simulink model "oldMLpendubotSimulink"  (R2024b)
settings: Solver=FixedStepAuto  StartTime=0.0  StopTime=10  FixedStep=dt  RelTol=1e-3
InitFcn:
  | simpb_init
values from neighbouring files (symbols this model uses):
  dt = 0.01    [EKF_stateFNpb.m]    (also in downrighttest.m = 0.001; pendubot_lqr.m; simpb_init.m)
  eqb = [-pi/2;0;0;0]    [downrighttest.m]    (also in pendubot_lqr.m = [pi/2;0;0;0]; simpb_init.m = [pi/2;0;0;0])
  mNoise = diag([mvar,mvar])    [downrighttest.m]    (also in simpb_init.m)
  mvar = 1e-3    (= 0.001)    [downrighttest.m]    (also in simpb_init.m = 0.0001)
  pNoise = diag([pvar,pvar,pvar,pvar])    [downrighttest.m]    (also in simpb_init.m)
  pvar = 0    [downrighttest.m]    (also in simpb_init.m = 1e-06)
  Q = diag([15,15,1,1])    [downrighttest.m]    (also in pendubot_lqr.m = diag([10,10,1,1]); simpb_init.m = diag([150,250,100,200]))
  q1dref = interp1(t_ref, q1dref, t_sim, 'pchip')    [pendubot_lqr.m]    (also in simpb_init.m)
  q1ref = interp1(t_ref, q1ref, t_sim, 'pchip')    [pendubot_lqr.m]    (also in simpb_init.m)
  q2dref = interp1(t_ref, q2dref, t_sim, 'pchip')    [pendubot_lqr.m]    (also in simpb_init.m)
  q2ref = interp1(t_ref, q2ref, t_sim, 'pchip')    [pendubot_lqr.m]    (also in simpb_init.m)
  R = 50    [downrighttest.m]    (also in pendubot_lqr.m = 5; simpb_init.m)
  uref = interp1(t_ref, uref, t_sim, 'pchip')    [pendubot_lqr.m]    (also in simpb_init.m)
  x0 = [-pi/4;0;0;0]    [downrighttest.m]    (also in pendubot_lqr.m = [-pi/2;0;0;0])
libraries: sharedTrackingLibrary x1
settings Model: Creator=heeirthan  LastModifiedBy=heeirthan

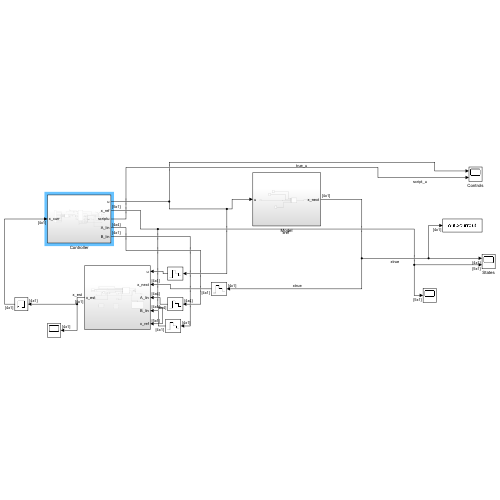
[thumbnail: Simulink's stored preview of the top-level diagram]
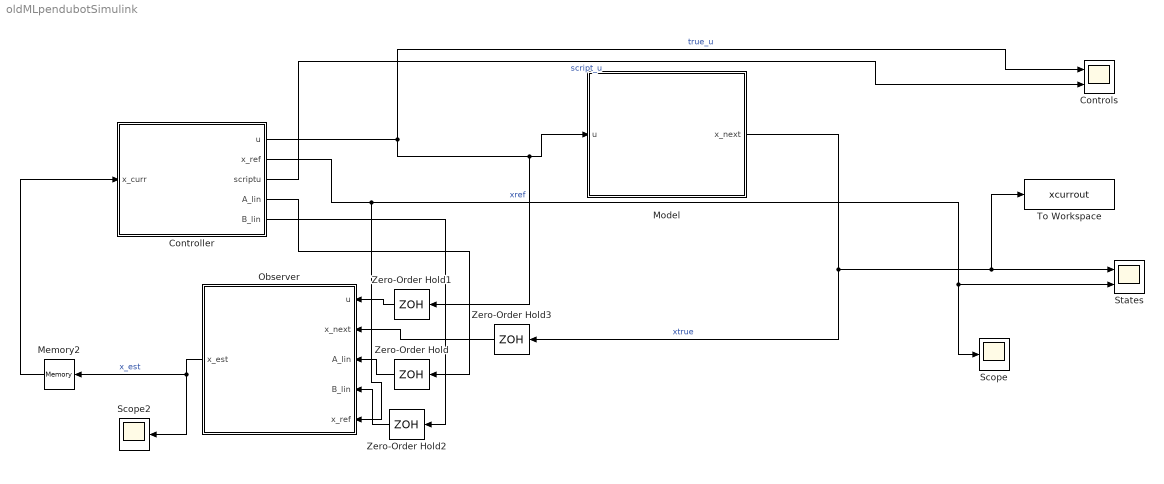
== system oldMLpendubotSimulink ==
  Controller : Subsystem
  Controls : Scope  NumInputPorts=2
  Memory2 : Memory  InitialCondition=x0
  Model : Subsystem
  Observer : Subsystem
  Scope : Scope
  Scope2 : Scope
  States : Scope  NumInputPorts=2
  To Workspace : ToWorkspace  VariableName=xcurrout  SaveFormat=Timeseries  SampleTime=-1
  Zero-Order Hold{,1..3} (4 alike) : ZeroOrderHold  SampleTime=dt
  wires:
  Observer/1(x_est) -> Memory2/1, Scope2/1  "x_est"
  Model/1(x_next) -> Zero-Order Hold3/1, To Workspace/1, States/1  "xtrue"
  Controller/2(x_ref) -> Observer/5(x_ref), Scope/1, States/2  "xref"
  Controller/3(scriptu) -> Controls/2  "script_u"
  Controller/1(u) -> Controls/1, Zero-Order Hold1/1, Model/1(u)  "true_u"
  Zero-Order Hold2/1 -> Observer/4(B_lin)
  Zero-Order Hold1/1 -> Observer/1(u)
  Zero-Order Hold3/1 -> Observer/2(x_next)
  Controller/4(A_lin) -> Zero-Order Hold/1
  Controller/5(B_lin) -> Zero-Order Hold2/1
  Memory2/1 -> Controller/1(x_curr)
  Zero-Order Hold/1 -> Observer/3(A_lin)

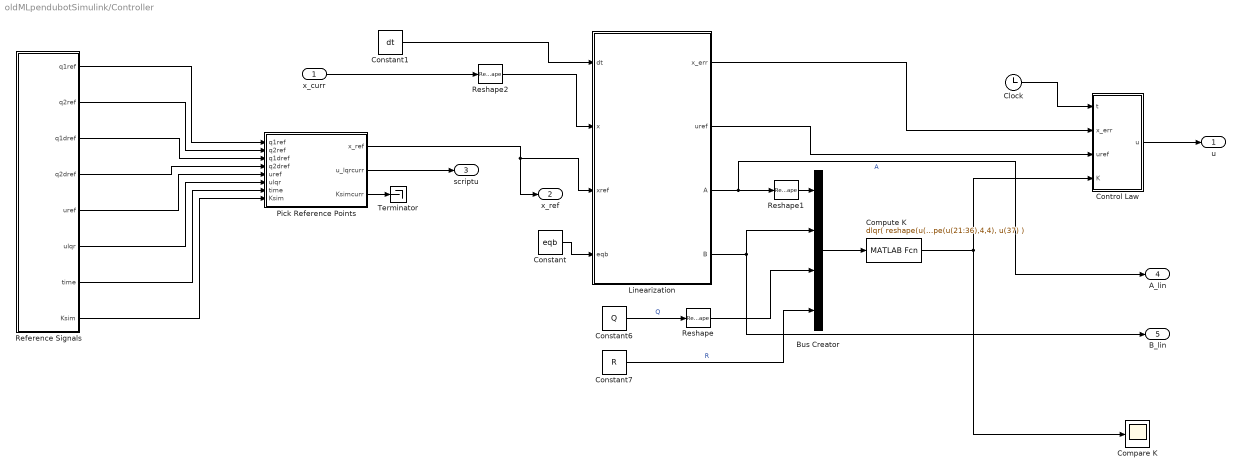
== system oldMLpendubotSimulink/Controller ==
  x_curr : Inport
  Bus Creator : BusCreator  Inputs=4
  Clock : Clock
  Compare K : Scope
  Compute K : MATLABFcn  MATLABFcn=dlqr( reshape(u(1:16),4,4), reshape(u(17:20),4,1), reshape(u(21:36),4,4), u(37) )  OutputDimensions=[1,4]  Output1D=off
  Constant : Constant  Value=eqb
  Constant1 : Constant  Value=dt
  Constant6 : Constant  Value=Q  SampleTime=-1
  Constant7 : Constant  Value=R  SampleTime=-1
  Control Law : MATLAB Function  TreatAsAtomicUnit=on
  Linearization : MATLAB Function  TreatAsAtomicUnit=on
  Pick Reference Points : MATLAB Function  TreatAsAtomicUnit=on
  Reference Signals : Subsystem
  Reshape : Reshape
  Reshape1 : Reshape
  Reshape2 : Reshape  OutputDimensionality=Customize  OutputDimensions=[4,1]
  Terminator : Terminator
  u : Outport
  x_ref : Outport  Port=2
  scriptu : Outport  Port=3
  A_lin : Outport  Port=4
  B_lin : Outport  Port=5
  wires:
  x_curr/1 -> Reshape2/1
  Pick Reference Points/1(x_ref) -> x_ref/1, Linearization/3(xref)
  Constant/1 -> Linearization/4(eqb)
  Linearization/3(A) -> A_lin/1, Reshape1/1  "A"
  Linearization/4(B) -> Bus Creator/2, B_lin/1
  Constant6/1 -> Reshape/1  "Q"
  Constant7/1 -> Bus Creator/4  "R"
  Bus Creator/1 -> Compute K/1
  Compute K/1 -> Compare K/1, Control Law/4(K)
  Control Law/1(u) -> u/1
  Reshape/1 -> Bus Creator/3
  Reshape1/1 -> Bus Creator/1
  Linearization/2(uref) -> Control Law/3(uref)
  Linearization/1(x_err) -> Control Law/2(x_err)
  Reshape2/1 -> Linearization/2(x)
  Pick Reference Points/2(u_lqrcurr) -> scriptu/1
  Reference Signals/8(Ksim) -> Pick Reference Points/8(Ksim)
  Reference Signals/1(q1ref) -> Pick Reference Points/1(q1ref)
  Reference Signals/2(q2ref) -> Pick Reference Points/2(q2ref)
  Reference Signals/3(q1dref) -> Pick Reference Points/3(q1dref)
  Reference Signals/4(q2dref) -> Pick Reference Points/4(q2dref)
  Reference Signals/5(uref) -> Pick Reference Points/5(uref)
  Reference Signals/6(ulqr) -> Pick Reference Points/6(ulqr)
  Reference Signals/7(time) -> Pick Reference Points/7(time)
  Clock/1 -> Control Law/1(t)
  Pick Reference Points/3(Ksimcurr) -> Terminator/1
  Constant1/1 -> Linearization/1(dt)

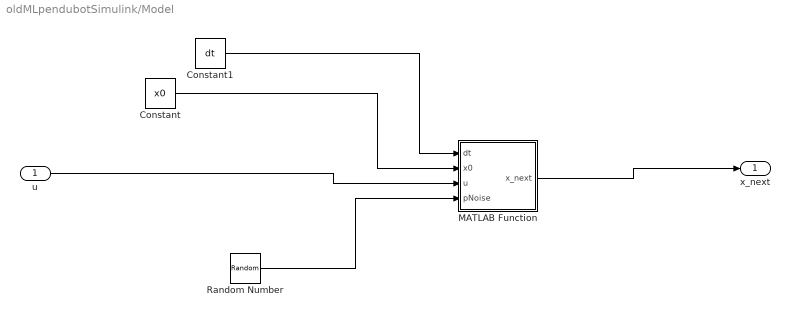
== system oldMLpendubotSimulink/Model ==
  u : Inport
  Constant : Constant  Value=x0
  Constant1 : Constant  Value=dt
  MATLAB Function : MATLAB Function  TreatAsAtomicUnit=on
  Random Number : RandomNumber  Variance=pvar  SampleTime=dt
  x_next : Outport
  wires:
  u/1 -> MATLAB Function/3(u)
  MATLAB Function/1(x_next) -> x_next/1
  Constant/1 -> MATLAB Function/2(x0)
  Random Number/1 -> MATLAB Function/4(pNoise)
  Constant1/1 -> MATLAB Function/1(dt)

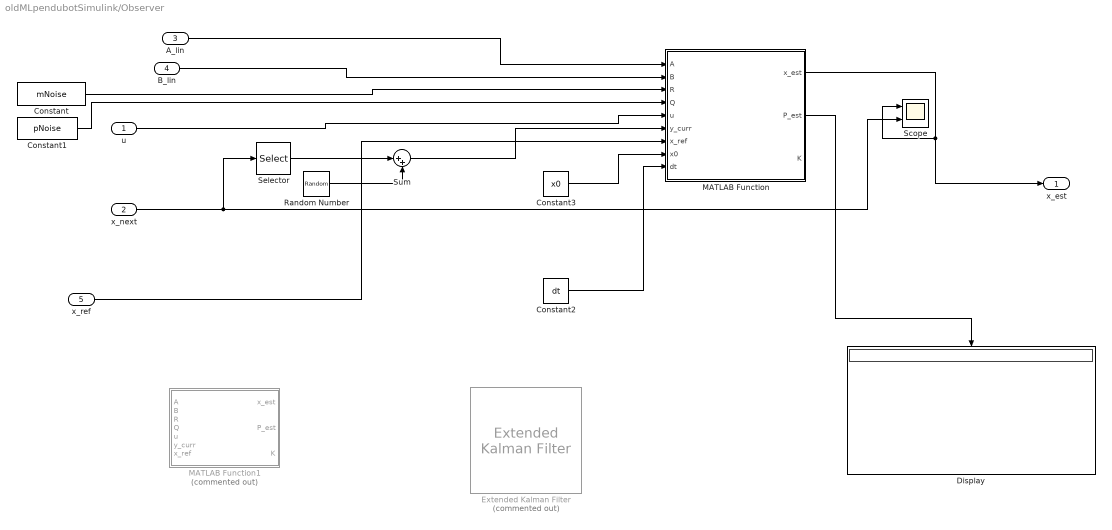
== system oldMLpendubotSimulink/Observer ==
  u : Inport
  x_next : Inport  Port=2
  A_lin : Inport  Port=3
  B_lin : Inport  Port=4
  x_ref : Inport  Port=5
  Constant : Constant  Value=mNoise
  Constant1 : Constant  Value=pNoise
  Constant2 : Constant  Value=dt
  Constant3 : Constant  Value=x0
  Display : Display
  Extended Kalman Filter : sharedTrackingLibrary/Extended Kalman Filter  Commented=on  StateTransitionFcn=EKF_stateFNpb  HasStateTransitionJacobianFcn=off  HasAdditiveProcessNoise=Additive  ProcessNoise=pNoise  HasTimeVaryingProcessNoise=off  HasStateTransitionFcnExtraArgument=1  InitialState=x0  InitialStateCovariance=initvar  MeasurementFcn1=measurementFcn  HasMeasurementJacobianFcn1=off  HasMeasurementEnablePort1=off  HasAdditiveMeasurementNoise1=Additive  MeasurementNoise1=mNoise  HasTimeVaryingMeasurementNoise1=off  HasMeasurementFcnExtraArgument1=0  HasMeasurementWrapping1=off  MeasurementFcn2=myMeasurementFcn  HasMeasurementJacobianFcn2=off  HasMeasurementEnablePort2=off  HasAdditiveMeasurementNoise2=Additive  MeasurementNoise2=1  HasTimeVaryingMeasurementNoise2=off  HasMeasurementFcnExtraArgument2=0  HasMeasurementWrapping2=off  MeasurementFcn3=myMeasurementFcn  HasMeasurementJacobianFcn3=off  HasMeasurementEnablePort3=off  HasAdditiveMeasurementNoise3=Additive  MeasurementNoise3=1  HasTimeVaryingMeasurementNoise3=off  HasMeasurementFcnExtraArgument3=0  HasMeasurementWrapping3=off  MeasurementFcn4=myMeasurementFcn  HasMeasurementJacobianFcn4=off  HasMeasurementEnablePort4=off  HasAdditiveMeasurementNoise4=Additive  MeasurementNoise4=1  HasTimeVaryingMeasurementNoise4=off  HasMeasurementFcnExtraArgument4=0  HasMeasurementWrapping4=off  MeasurementFcn5=myMeasurementFcn  HasMeasurementJacobianFcn5=off  HasMeasurementEnablePort5=off  HasAdditiveMeasurementNoise5=Additive  MeasurementNoise5=1  HasTimeVaryingMeasurementNoise5=off  HasMeasurementFcnExtraArgument5=0  HasMeasurementWrapping5=off  EnableMultirate=off  StateTransitionFcnSampleTime=1  MeasurementFcn1SampleTime=1  MeasurementFcn2SampleTime=1  MeasurementFcn3SampleTime=1  MeasurementFcn4SampleTime=1  MeasurementFcn5SampleTime=1  UseCurrentEstimator=on  OutputStateCovariance=on  DataType=double  SampleTime=dt  NumberOfMeasurements=1
  MATLAB Function : MATLAB Function  TreatAsAtomicUnit=on
  MATLAB Function1 : MATLAB Function  Commented=on  TreatAsAtomicUnit=on
  Random Number : RandomNumber  Variance=mvar  SampleTime=dt
  Scope : Scope  NumInputPorts=2
  Selector : Selector  InputPortWidth=4  IndexOptions=Index vector (dialog)  Indices=[1 2]  OutputSizes=1
  Sum : Sum  Inputs=|++
  x_est : Outport
  wires:
  x_next/1 -> Scope/2, Selector/1
  Selector/1 -> Sum/1
  Random Number/1 -> Sum/2
  MATLAB Function/1(x_est) -> x_est/1, Scope/1
  Constant/1 -> MATLAB Function/3(R)
  Constant1/1 -> MATLAB Function/4(Q)
  Sum/1 -> MATLAB Function/6(y_curr)
  A_lin/1 -> MATLAB Function/1(A)
  B_lin/1 -> MATLAB Function/2(B)
  u/1 -> MATLAB Function/5(u)
  Constant3/1 -> MATLAB Function/8(x0)
  Constant2/1 -> MATLAB Function/9(dt)
  x_ref/1 -> MATLAB Function/7(x_ref)
  MATLAB Function/2(P_est) -> Display/1

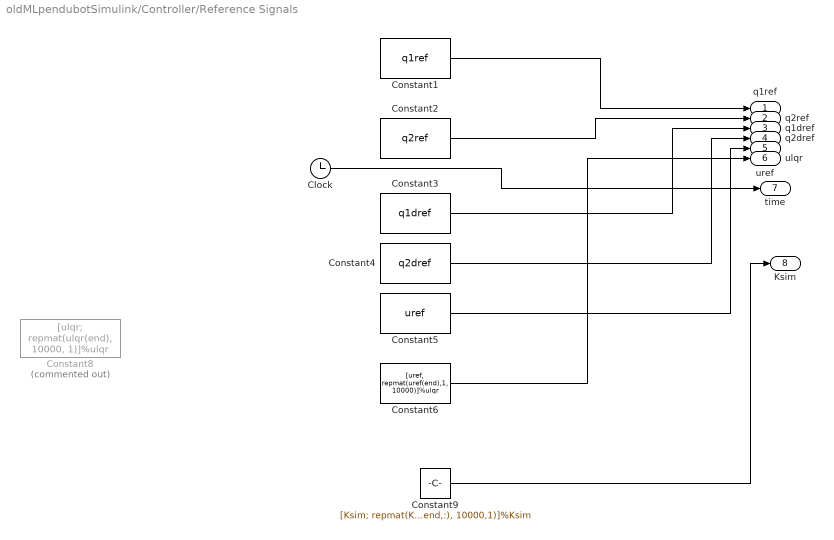
== system oldMLpendubotSimulink/Controller/Reference Signals ==
  Clock : Clock
  Constant1 : Constant  Value=q1ref  SampleTime=-1
  Constant2 : Constant  Value=q2ref  SampleTime=-1
  Constant3 : Constant  Value=q1dref  SampleTime=-1
  Constant4 : Constant  Value=q2dref  SampleTime=-1
  Constant5 : Constant  Value=uref  SampleTime=-1
  Constant6 : Constant  Value=[uref, repmat(uref(end),1, 10000)]%ulqr  SampleTime=-1
  Constant8 : Constant  Commented=on  Value=[ulqr; repmat(ulqr(end), 10000, 1)]%ulqr  SampleTime=-1
  Constant9 : Constant  Value=[Ksim; repmat(Ksim(end,:), 10000,1)]%Ksim
  q1ref : Outport
  q2ref : Outport  Port=2
  q1dref : Outport  Port=3
  q2dref : Outport  Port=4
  uref : Outport  Port=5
  ulqr : Outport  Port=6
  time : Outport  Port=7
  Ksim : Outport  Port=8
  wires:
  Constant1/1 -> q1ref/1
  Constant6/1 -> ulqr/1
  Clock/1 -> time/1
  Constant5/1 -> uref/1
  Constant3/1 -> q1dref/1
  Constant4/1 -> q2dref/1
  Constant2/1 -> q2ref/1
  Constant9/1 -> Ksim/1

== matlab function oldMLpendubotSimulink/Model/MATLAB Function ==
  data: dt input; x0 input; u input; x_next output; pNoise input
function x_next = fcn(dt, x0, u, pNoise)

%From REal pendulum in lab
p.theta1 = 0.0308; 
p.theta2 = 0.0106;
p.theta3 = 0.0095;
p.theta4 = 0.2087;
p.theta5 = 0.063;
p.g = 9.8;

persistent x;
if isempty(x)
    x = x0;
end

x_next = rk4_step(@(xx, uu) dx_pb_lqrreal(0,xx, uu, p), x, u,dt);
x_next(1) = wrapToPi(x_next(1));
x_next(2) = wrapToPi(x_next(2));

x_next = x_next + pNoise;
x = x_next;
end

== matlab function oldMLpendubotSimulink/Controller/Linearization ==
  data: dt input; x_err output; uref output; x input; A output; xref input; eqb input; B output
function [x_err, uref, A,B]  = fcn(dt,x,xref, eqb)


q1ref = xref(1);
q2ref = xref(2);
q1dref = xref(3);
q2dref = xref(4);
uref = xref(5);

norm([x(1);x(2)]-[pi/2;0])
%Linearize about ref/equilibrium
if (norm([x(1);x(2)]-[pi/2;0]) > -0.3)
    %Linearize about current ref traj
    A = Afunfile(q1ref, q2ref, q1dref, q2dref, uref);
    B = Bfunfile(q1ref, q2ref, q1dref, q2dref, uref);
    
    x_err = [wrapToPi(x(1)-q1ref);
    wrapToPi(x(2)-q2ref);
    x(3) - q1dref;
    x(4)-q2dref];
else
    disp('In second controller')
    
    A = Afunfile(eqb(1), eqb(2), eqb(3), eqb(4), 0);
    B = Bfunfile(eqb(1), eqb(2), eqb(3), eqb(4), 0);

    x_err = [wrapToPi(x(1)-eqb(1));
    wrapToPi(x(2)-eqb(2));
    x(3) - eqb(3);
    x(4)-eqb(4)];
end


% Euler discretize here
A = eye(4) + dt*A;
B = dt * B;

== matlab function oldMLpendubotSimulink/Controller/Pick Reference Points ==
  data: x_ref output; q1ref input; q2ref input; q1dref input; q2dref input; uref input; ulqr input; u_lqrcurr output; time input; Ksim input; Ksimcurr output
function [x_ref,u_lqrcurr, Ksimcurr] = fcn(q1ref,q2ref,q1dref,q2dref, uref, ulqr, time,Ksim)

persistent t;
if isempty(t)
    t = 1;
else 
    t = t+1;
end

t
if t > length(q1ref)
    x_ref = [pi/2;0;0;0;0];
else    
    x_ref = [q1ref(t);q2ref(t);q1dref(t);q2dref(t);uref(t)];
    
end
u_lqrcurr = ulqr(t); %not used, just for plotting
Ksimcurr = Ksim(t,:);

== matlab function oldMLpendubotSimulink/Controller/Control Law ==
  data: t input; x_err input; uref input; K input; u output
function u = fcn(t, x_err,uref,K)
persistent K_prev;
if isempty(K_prev)
    K_prev = [0,0,0,0];
end
K
mk = max(abs(K));
if ~all(K_prev == 0)
    if (K(3) > 5 || K(3) < -7)
        K(3) = K_prev(3);
    end
    if (K(4) > 5 || K(4) < -7)
        K(4) = K_prev(4);
    end
    if (K(1) > 0 || K(1) < -34)
        K(1) = K_prev(1);
    end
    if (K(2) > 0 || K(2) < -34)
        K(2) = K_prev(2);
    end
end
K
% if t > 1.4 - 0.3 && t < 1.4 + 0.6
%     K = K_prev;
%     disp('Using prev K')
% end
u = uref - K * x_err;
u_max = 10;
u = max(-u_max, min(u,u_max));
K_prev = K;

== matlab function oldMLpendubotSimulink/Observer/MATLAB Function ==
  data: A input; B input; R input; Q input; u input; y_curr input; x_est output; P_est output; K output; x_ref input; x0 input; dt input
function [x_est, P_est, K] = extended_kalman_filter(A, B,R, Q, u, y_curr, x_ref, x0, dt)
persistent x;
if isempty(x)
    x = x0;
end
persistent P;
if isempty(P)
    P = eye(4)*1e-6;
end

%From REal pendulum in lab
p.theta1 = 0.0308; 
p.theta2 = 0.0106;
p.theta3 = 0.0095;
p.theta4 = 0.2087;
p.theta5 = 0.063;
p.g = 9.8;

xr = x_ref(1:4);

C = [1 0 0 0;
    0 1 0 0];

dt = 0.01;
x_pred = rk4_step(@(xx, uu) dx_pb_lqrreal(0,xx, uu, p), x, u,dt);
%x_pred(1) = wrapToPi(1);
%x_pred(2) = wrapToPi(2);
A = Afunfile(x(1),x(2),x(3),x(4),u);

%P_pred = A*P*A' + Q;
P_pred = A*P*A' + Q;
%P_est = P_pred;
% for n=1:1000
%     P_pred = A*P_est*A' + Q;
%     K = (P_pred*C') * (C * P_pred * C' + R)^(-1);
%     P_est = (eye(4) - K*C) * P_pred * (eye(4) - K*C)' + K*R*K';
% end

K = (P_pred * C') * (C*P_pred*C' + R)^-1;
x_est = x_pred + K*(y_curr - C*x_pred);
P_est = ((eye(4)-K*C) * P_pred * (eye(4)-K*C)' + K*R*K');
 
x_est(1) = wrapToPi(x_est(1));
x_est(2) = wrapToPi(x_est(2));
x = x_est;
P = P_est;

== matlab function oldMLpendubotSimulink/Observer/MATLAB Function1 ==
  data: A input; B input; R input; Q input; u input; y_curr input; x_est output; P_est output; K output; x_ref input
function [x_est, P_est, K] = kalman_filter(A, B,R, Q, u, y_curr, x_ref)
persistent x;
if isempty(x)
    x = [-pi/2;0;0;0];
end
persistent P;
if isempty(P)
    P = eye(4)*1e-6;
end

xr = x_ref(1:4);

C = [1 0 0 0;
    0 1 0 0];

x_pred = A*(x-xr) + xr + B*(u - x_ref(5)); %error + xref
%x_pred(1) = wrapToPi(1);
%x_pred(2) = wrapToPi(2);
P_pred = A*P*A' + Q;
P_est = P_pred;
for n=1:1000
    P_pred = A*P_est*A' + Q;
    K = (P_pred*C') * (C * P_pred * C' + R)^(-1);
    P_est = (eye(4) - K*C) * P_pred * (eye(4) - K*C)' + K*R*K';
end

%K = (P_pred * C') * (C*P_pred*C' + R)^-1;
x_est = x_pred + K*(y_curr - C*x_pred);
%P_est = ((eye(4)-K*C) * P_pred * (eye(4)-K*C)' + K*R*K');
x_est(1) = wrapToPi(x_est(1));
x_est(2) = wrapToPi(x_est(2));
x = x_est;
P = P_est;
